simulink model "qpsk"  (Simulink 7.6)
settings: Solver=ode45  StartTime=0.0  StopTime=200  RelTol=1e-3
undefined symbols (not defined in the file): j
libraries: dsp_blocks x7, simulink x2
settings Model: Creator=Joshan  LastModifiedBy=Joshan

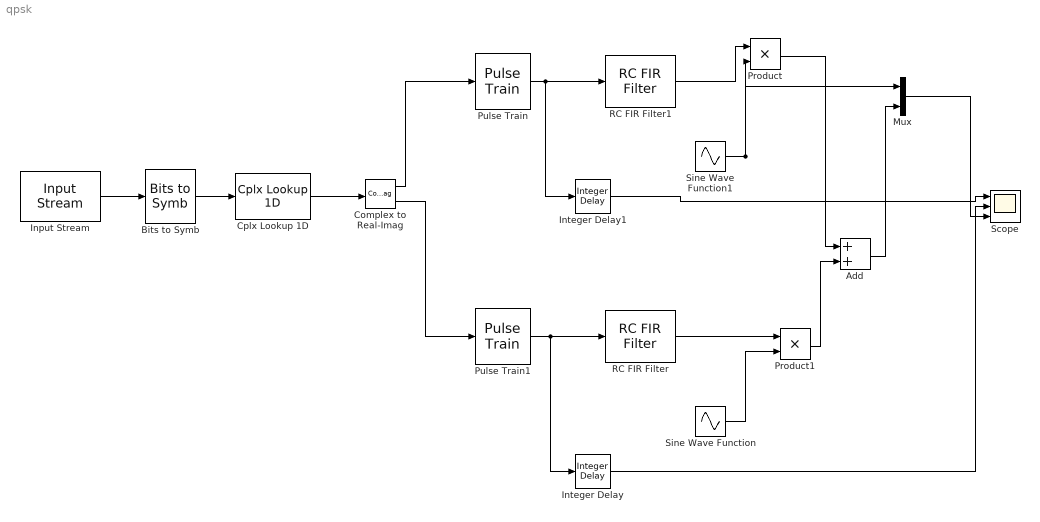
== system qpsk ==
  Add : Sum
  Bits to Symb : dsp_blocks/Conversions/Bits to Symb  SystemSampleTime=-1
  Complex to Real-Imag : ComplexToRealImag
  Cplx Lookup 1D : dsp_blocks/Conversions/Cplx Lookup 1D  SystemSampleTime=-1  table=[1 j -1 -j]
  Input Stream : dsp_blocks/Sources//Sinks/Input Stream  SystemSampleTime=-1  period=50  width=2  fname=rand.mat
  Integer Delay : simulink/Discrete/Integer Delay  NumDelays=64  vinit=0.0  samptime=-1
  Integer Delay1 : simulink/Discrete/Integer Delay  NumDelays=64  vinit=0.0  samptime=-1
  Mux : Mux  Inputs=2
  Product : Product  RndMeth=Zero
  Product1 : Product  RndMeth=Zero
  Pulse Train : dsp_blocks/Conversions/Pulse Train  SystemSampleTime=-1  period=10
  Pulse Train1 : dsp_blocks/Conversions/Pulse Train  SystemSampleTime=-1  period=10
  RC FIR Filter : dsp_blocks/Filters/RC FIR Filter  SystemSampleTime=-1  period=10  beta=0.5  root=off  filt_len=128  win_type=off
  RC FIR Filter1 : dsp_blocks/Filters/RC FIR Filter  SystemSampleTime=-1  period=10  beta=0.5  root=off  filt_len=128  win_type=off
  Scope : Scope  NumInputPorts=3
      settings: TimeRange=0.8045052292839898  YMin=-2~-2~0.9202072538860111  YMax=2~2~2.520207253886011
  Sine Wave Function : Sin  Amplitude=-1  Frequency=2*pi*0.1  SampleTime=0
  Sine Wave Function1 : Sin  Frequency=2*pi*0.1  Phase=pi/2  SampleTime=0
  wires:
  Input Stream/1 -> Bits to Symb/1
  Bits to Symb/1 -> Cplx Lookup 1D/1
  Cplx Lookup 1D/1 -> Complex to Real-Imag/1
  Complex to Real-Imag/1 -> Pulse Train/1
  Complex to Real-Imag/2 -> Pulse Train1/1
  Pulse Train1/1 -> RC FIR Filter/1, Integer Delay/1
  Pulse Train/1 -> RC FIR Filter1/1, Integer Delay1/1
  RC FIR Filter/1 -> Product1/1
  RC FIR Filter1/1 -> Product/1
  Sine Wave Function/1 -> Product1/2
  Sine Wave Function1/1 -> Product/2, Mux/1
  Integer Delay1/1 -> Scope/1
  Integer Delay/1 -> Scope/2
  Product1/1 -> Add/2
  Add/1 -> Mux/2
  Mux/1 -> Scope/3
  Product/1 -> Add/1
